simulink model "modelo_state_space"  (Simulink 8.5)
settings: Solver=ode45  StartTime=0.0  StopTime=ttotal  MaxStep=1e-2  RelTol=1e-8
values from neighbouring files (symbols this model uses):
  A = [0 1 ; a1 a2]    [e_12.m]    (also in e_13.m; e_8.m; e_9.m; lab3.m)
  B = [0;  1/J]    [e_12.m]    (also in e_13.m; e_8.m; e_9.m; lab3.m)
  C = [1 0]    [e_12.m]    (also in e_13.m = [1 0; 0 1]; e_8.m = [1 0; 0 1]; e_9.m = [1 0; 0 1]; lab3.m = [1 0; 0 1])
  T = T_v(n)    [e_11.m]    (also in e_13.m = 0; e_8.m = 0; e_9.m = 0; lab3.m = 0)
  x0 = [pi/4 0]    [e_13.m]    (also in e_8.m = vec_prop(:,n); e_9.m; lab3.m; lab3_1.m = [0 pi/4])
settings Model: Creator=ines-  LastModifiedBy=ricar
settings DataIOCC: SignalLoggingSaveFormat=Dataset
settings OptimizationCC: ExpressionDepthLimit=128
settings DebuggingCC: UnderspecifiedInitializationDetection=Simplified  MergeDetectMultiDrivingBlocksExec=error  FcnCallInpInsideContextMsg=EnableAllAsError  StateNameClashWarn=none
settings GRTTargetCC: CombineOutputUpdateFcns=on  GRTInterface=off

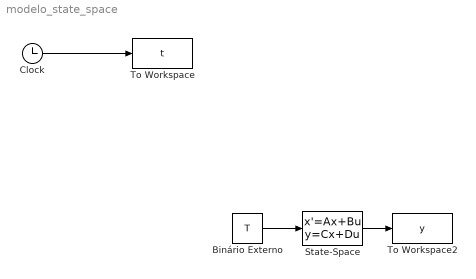
== system modelo_state_space ==
  Binário Externo : Constant  Value=T
  Clock : Clock
  State-Space : StateSpace  A=A  B=B  C=C  D=[0; 0]  X0=x0
  "To Workspace  " : ToWorkspace  VariableName=t  SampleTime=-1
  To Workspace2 : ToWorkspace  VariableName=y  SampleTime=-1
  wires:
  Clock/1 -> "To Workspace  "/1
  State-Space/1 -> To Workspace2/1
  Binário Externo/1 -> State-Space/1
